simulink model "v1"  (R2025b)
settings: Solver=VariableStepAuto  StartTime=0.0  StopTime=10.0  RelTol=1e-3
libraries: simulink x4, fuzblock x1
settings Model: Creator=DELL  LastModifiedBy=DELL

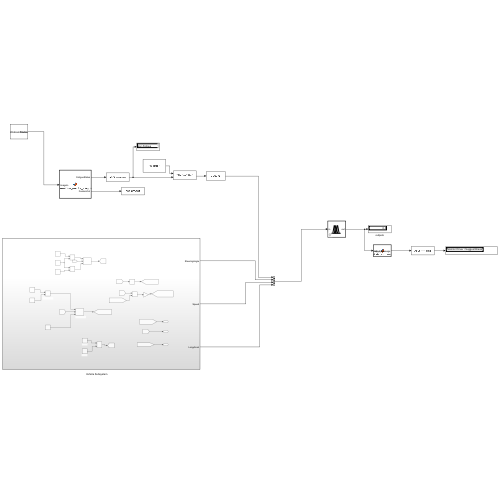
[thumbnail: Simulink's stored preview of the top-level diagram]
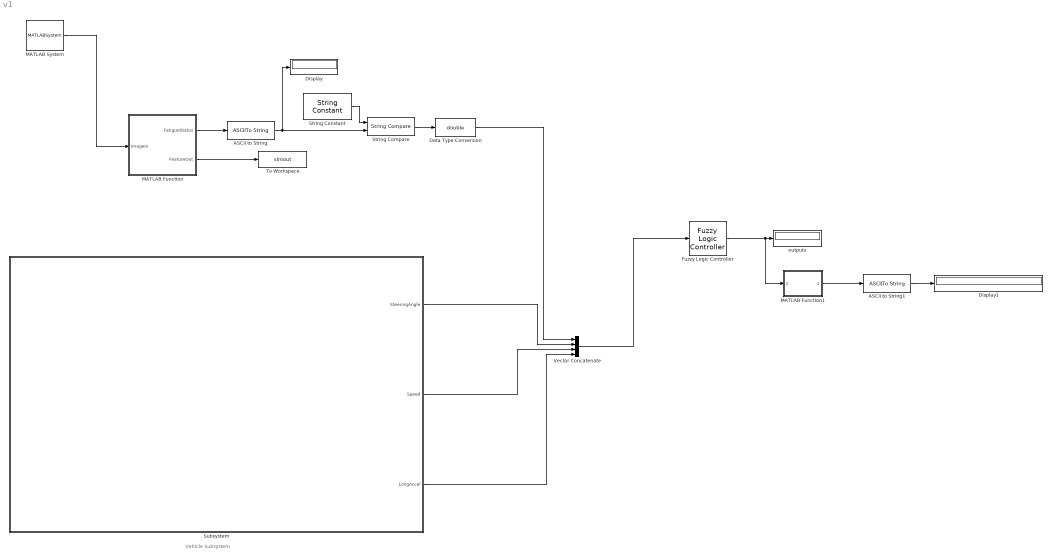
== system v1 ==
  note: Vehicle Subsystem
  ASCII to String : ASCIIToString
  ASCII to String1 : ASCIIToString
  Data Type Conversion : DataTypeConversion  OutDataTypeStr=double  SaturateOnIntegerOverflow=off  RndMeth=Floor
  Display : Display
  Display1 : Display
  Fuzzy Logic Controller : fuzblock/Fuzzy Logic  Controller  FIS=FinalDrowsinessRisk  OutputSampleNumber=101  DataType=double  UseLookupTable=off  NumBreakpoints=10  FuzzifiedInputs=off  RuleFiringStrengths=off  RuleOutputs=off  AggregatedOutputs=off  SimulateUsing=Interpreted execution  OutOfRangeInputValueMessage=warning  NoRuleFiredMessage=warning  EmptyOutputFuzzySetMessage=warning
  MATLAB Function : MATLAB Function  TreatAsAtomicUnit=on
  MATLAB Function1 : MATLAB Function  TreatAsAtomicUnit=on
  MATLAB System : MATLABSystem  System=WebcamSource  SimulateUsing=Interpreted execution
      mask Type: WebcamSource
  String Compare : StringCompare
  String Constant : StringConstant  String="\"Fatigue\""
  Subsystem : Subsystem
  To Workspace : ToWorkspace  VariableName=simout  SaveFormat=Timeseries  SampleTime=-1
  Vector Concatenate : Concatenate  NumInputs=4
  outputs : Display
  wires:
  MATLAB System/1 -> MATLAB Function/1(ImageIn)
  MATLAB Function/2(FeatureOut) -> To Workspace/1
  MATLAB Function/1(FatigueStatus) -> ASCII to String/1
  ASCII to String/1 -> String Compare/2, Display/1
  Vector Concatenate/1 -> Fuzzy Logic Controller/1
  Fuzzy Logic Controller/1 -> MATLAB Function1/1(risk_score), outputs/1
  String Constant/1 -> String Compare/1
  String Compare/1 -> Data Type Conversion/1
  Data Type Conversion/1 -> Vector Concatenate/1
  Subsystem/1(SteeringAngle) -> Vector Concatenate/2
  Subsystem/2(Speed) -> Vector Concatenate/3
  Subsystem/3(LongAccel) -> Vector Concatenate/4
  MATLAB Function1/1(output_message) -> ASCII to String1/1
  ASCII to String1/1 -> Display1/1

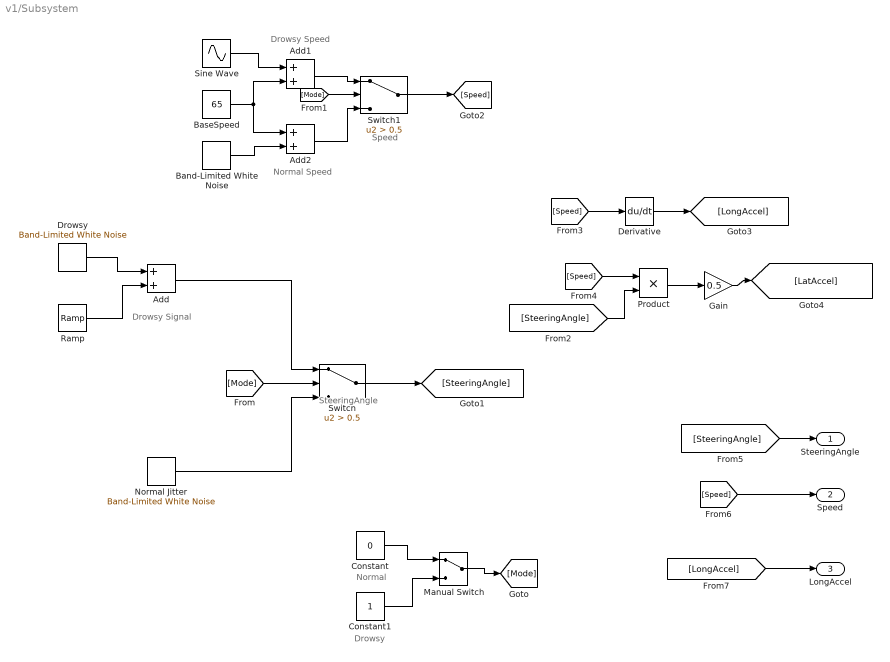
== system v1/Subsystem ==
  note: SteeringAngle
  note: Speed
  note: Drowsy Signal
  note: Drowsy
  note: Normal
  note: Drowsy Speed
  note: Normal Speed
  Add : Sum
  Add1 : Sum
  Add2 : Sum
  Band-Limited White Noise : simulink/Sources/Band-Limited White Noise  Cov=[0.01]  Ts=0.01  seed=[23341]
  BaseSpeed : Constant  Value=65
  Constant : Constant  Value=0
  Constant1 : Constant
  Derivative : Derivative
  Drowsy : simulink/Sources/Band-Limited White Noise  Cov=[0.1]  Ts=0.01  seed=[23341]
  Gain : Gain  Gain=0.5
  Manual Switch : ManualSwitch
  Normal Jitter : simulink/Sources/Band-Limited White Noise  Cov=[0.001]  Ts=0.01  seed=[23341]
  Product : Product
  Ramp : simulink/Sources/Ramp  slope=0.005  start=0  InitialOutput=0
  Sine Wave : Sin  Amplitude=8  Frequency=0.05  SampleTime=0.01
  Switch : Switch  Criteria=u2 > Threshold  Threshold=0.5  SaturateOnIntegerOverflow=off  InputSameDT=off
  Switch1 : Switch  Criteria=u2 > Threshold  Threshold=0.5  SaturateOnIntegerOverflow=off  InputSameDT=off
  SteeringAngle : Outport
  Speed : Outport  Port=2
  LongAccel : Outport  Port=3
  wires:
  Constant/1 -> Manual Switch/1
  Constant1/1 -> Manual Switch/2
  Manual Switch/1 -> [Mode]
  Drowsy/1 -> Add/1
  Ramp/1 -> Add/2
  [Mode] -> Switch/2
  Add/1 -> Switch/1
  Normal Jitter/1 -> Switch/3
  Sine Wave/1 -> Add1/1
  BaseSpeed/1 -> Add2/1, Add1/2
  Band-Limited White Noise/1 -> Add2/2
  Add1/1 -> Switch1/1
  Add2/1 -> Switch1/3
  [Mode] -> Switch1/2
  Derivative/1 -> [LongAccel]
  Switch/1 -> [SteeringAngle]
  Product/1 -> Gain/1
  Gain/1 -> [LatAccel]
  Switch1/1 -> [Speed]
  [SteeringAngle] -> Product/2
  [Speed] -> Derivative/1
  [Speed] -> Product/1
  [SteeringAngle] -> SteeringAngle/1
  [Speed] -> Speed/1
  [LongAccel] -> LongAccel/1

== matlab function v1/MATLAB Function1 ==
  data: risk_score input; output_message output
function output_message = textual_decision_wrapper(risk_score)
    % Define the external function (required for code generation)
    coder.extrinsic('textual_decision');

    % Pre-allocate output size (MANDATORY: must match the size in textual_decision.m)
    output_message = zeros(1, 30, 'uint8');

    % Call the external function
    output_message = textual_decision(risk_score);
end

== matlab function v1/MATLAB Function ==
  data: FatigueStatus output; FeatureOut output; ImageIn input
function [FatigueStatus, FeatureOut] = drowsiness_monitor_wrapper(ImageIn)
% Define the external function
coder.extrinsic('detect_drowsiness_extrinsic');

% Pre-allocate outputs for Code Generation (MANDATORY)
FatigueStatus = zeros(1, 20, 'uint8');
FeatureOut = zeros(1, 4);

% Call the external function (runs in standard MATLAB)
[FatigueStatus, FeatureOut] = detect_drowsiness_extrinsic(ImageIn);

end
